simulink model "p_c"  (R2014b)
settings: Solver=ode3  StartTime=0.0  StopTime=simtime  FixedStep=0.01  RelTol=1e-3
values from neighbouring files (symbols this model uses):
  a = 1    [cosine_path_config.m]    (also in run.m = 0.4; run_alpha.m = 0.3; run_visual.m = 0.4)
  init_state = [-5;0.6*pi]    [run.m]    (also in run_visual.m)
  init_state_dot = [0;0]    [run.m]    (also in run_visual.m)
  w = pi/5    (= 0.628318530718)    [cosine_path_config.m]    (also in path_config.m = motion_parameters(1); run.m = 0.0628318530718; run_alpha.m; run_visual.m)
settings Model: Creator=Fredrik  LastModifiedBy=Fredrik

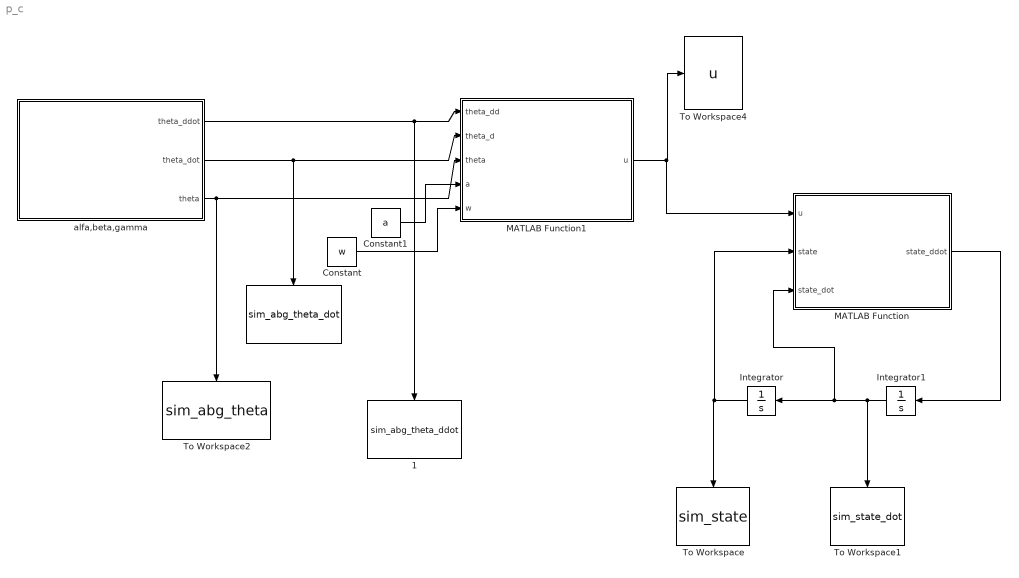
== system p_c ==
  " " : ToWorkspace  VariableName=sim_abg_theta_dot  SaveFormat=Structure With Time  SampleTime=-1
  " 1" : ToWorkspace  VariableName=sim_abg_theta_ddot  SaveFormat=Structure With Time  SampleTime=-1
  Constant : Constant  Value=w
  Constant1 : Constant  Value=a
  Integrator : Integrator  InitialCondition=init_state
  Integrator1 : Integrator  InitialCondition=init_state_dot
  MATLAB Function : MATLAB Function  TreatAsAtomicUnit=on
  MATLAB Function1 : MATLAB Function  TreatAsAtomicUnit=on
  To Workspace : ToWorkspace  VariableName=sim_state  SaveFormat=Structure With Time  SampleTime=-1
  To Workspace1 : ToWorkspace  VariableName=sim_state_dot  SaveFormat=Structure With Time  SampleTime=-1
  To Workspace2 : ToWorkspace  VariableName=sim_abg_theta  SaveFormat=Structure With Time  SampleTime=-1
  To Workspace4 : ToWorkspace  VariableName=u  SaveFormat=Structure With Time  SampleTime=-1
  "alfa,beta,gamma " : Subsystem
  wires:
  MATLAB Function/1(state_ddot) -> Integrator1/1
  Integrator1/1 -> Integrator/1, MATLAB Function/3(state_dot), To Workspace1/1
  Integrator/1 -> To Workspace/1, MATLAB Function/2(state)
  "alfa,beta,gamma "/3(theta) -> MATLAB Function1/3(theta), To Workspace2/1
  "alfa,beta,gamma "/2(theta_dot) -> MATLAB Function1/2(theta_d), " "/1
  "alfa,beta,gamma "/1("theta_ddot ") -> " 1"/1, MATLAB Function1/1(theta_dd)
  MATLAB Function1/1(u) -> MATLAB Function/1(u), To Workspace4/1
  Constant/1 -> MATLAB Function1/5(w)
  Constant1/1 -> MATLAB Function1/4(a)

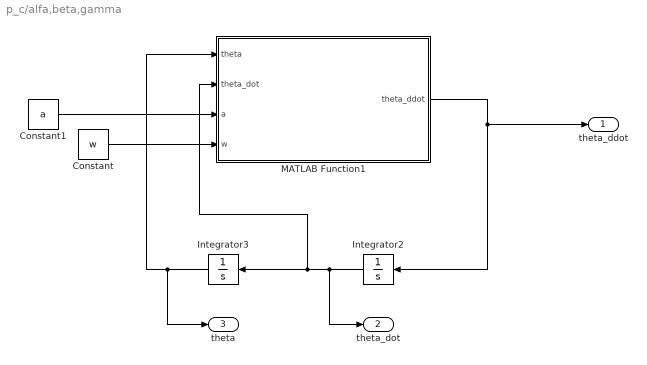
== system p_c/alfa,beta,gamma  ==
  Constant : Constant  Value=w
  Constant1 : Constant  Value=a
  Integrator2 : Integrator  InitialCondition=init_state_dot(2)
  Integrator3 : Integrator  InitialCondition=init_state(2)
  MATLAB Function1 : MATLAB Function  TreatAsAtomicUnit=on
  "theta_ddot " : Outport
  theta_dot : Outport  Port=2
  theta : Outport  Port=3
  wires:
  MATLAB Function1/1(theta_ddot) -> "theta_ddot "/1, Integrator2/1
  Integrator3/1 -> theta/1, MATLAB Function1/1(theta)
  Integrator2/1 -> theta_dot/1, Integrator3/1, MATLAB Function1/2(theta_dot)
  Constant/1 -> MATLAB Function1/4(w)
  Constant1/1 -> MATLAB Function1/3(a)

== matlab function p_c/alfa,beta,gamma /MATLAB Function1 ==
  data: theta input; theta_ddot output; theta_dot input; a input; w input
function theta_ddot  = fcn(theta, theta_dot, a, w)
%#codegen

%alfa=(cos(theta)*sin(theta/a))/(a*w*sqrt(sin(theta/a)^2)) - sin(theta)*cos(theta) + 1;
%beta=sin(theta)*cos(theta);
%gamma=-9.81*sin(theta);

g=9.81;

%verison1
alfa = cos(theta)*(-cos(theta)*sqrt(1-cos(theta/a)^2)*a*w+sin(theta/a))/(sqrt(1-cos(theta/a)^2)*a*w)+1;
beta= cos(theta)*sin(theta);
gamma=-g*sin(theta);


%version2
%alfa = cos(theta)*(-cos(theta)*sqrt(1-cos(theta/a)^2)*a*w-sin(theta/a))/(sqrt(1-cos(theta/a)^2)*a*w)+1;
%beta = cos(theta)*sin(theta);
%gamma = -g*sin(theta);


theta_ddot = (-beta*(theta_dot^2) - gamma)/alfa;

== matlab function p_c/MATLAB Function ==
  data: u input; state_ddot output size=2; state input size=2; state_dot input size=2
function state_ddot  = fcn(u,state, state_dot)



x = state(1);
theta = state(2);
x_dot = state_dot(1);
theta_dot = state_dot(2);
g = 9.81;



x_ddot = (1/(cos(theta)^2-2))*(g*sin(theta)*cos(theta) - u - sin(theta)*theta_dot^2);
theta_ddot = (1/(cos(theta)^2-2))*(-2*g*sin(theta) + u*cos(theta) + sin(theta)*cos(theta)*theta_dot^2);


state_ddot = [x_ddot; theta_ddot];

== matlab function p_c/MATLAB Function1 ==
  data: theta_dd input; theta_d input; u output; theta input; a input; w input
function u = fcn(theta_dd, theta_d, theta, a, w)

xc_dd=(sin(theta)*(theta_d)^2*sqrt(1-cos(theta/a)^2)*a*w-cos(theta)*(theta_dd)*sqrt(1-cos(theta/a)^2)*a*w+sin(theta/a)*(theta_dd))/(sqrt(1-cos(theta/a)^2)*a*w);

u=-(2*xc_dd + cos(theta)*theta_dd - sin(theta)*(theta_d^2));
